simulink library "energyEstimate"  (R2018a)
settings: Solver=VariableStepAuto  StartTime=0.0  StopTime=10.0  RelTol=1e-3
settings Model: Creator=mitch  LastModifiedBy=mitch

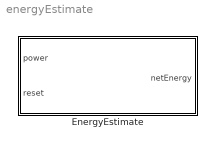
== system energyEstimate ==
  EnergyEstimate : Subsystem

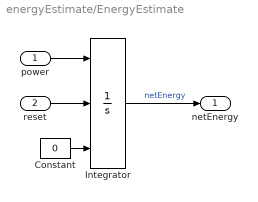
== system energyEstimate/EnergyEstimate ==
  power : Inport
  reset : Inport  Port=2  OutDataTypeStr=boolean
  Constant : Constant  Value=0
  Integrator : Integrator  ExternalReset=rising  InitialConditionSource=external
  netEnergy : Outport
  wires:
  reset/1 -> Integrator/2
  Constant/1 -> Integrator/3
  Integrator/1 -> netEnergy/1  "netEnergy"
  power/1 -> Integrator/1
